simulink model "harness"  (Simulink 7.0)
settings: Solver=ode23  StartTime=0.0  StopTime=20  FixedStep=0.01  RelTol=1e-3
InitFcn:
  | init_simulation
StopFcn:
  | post_simulation
values from neighbouring files (symbols this model uses):
  A = pi*R^2    (= 0.0506707479097)    [constants.m]
  accel_noise = noise_on*.01^2    [constants.m]
  Alpha = pi/180*[-85:5:85]    [constants.m]
  att_noise = noise_on*(.25*pi/180)^2    [constants.m]
  att_ref = [0.2 0.2 0 0 0 0]'    [run_simulation.m]
  att_traj_on = 0    [set_scenario.m]
  b = 0.1    [constants.m]
  const_wind = [1 1 0]    [run_simulation.m]
  g = [0 0 9.8]'    [constants.m]
  gyro_noise = noise_on*.01^2    [constants.m]
  J = [Jxx 0 0 ... (first row only)    [constants.m]
  K_a1s = .009    (= 0.009)    [constants.m]
  K_attitude = [  0   kp_p   kp_y     0    kd_p   kd_y ... (first row only)    [run_simulation.m]
  K_beta = 0.23    [constants.m]
  K_dz = 0.7    [run_simulation.m]
  K_flap = 4*(K_beta + T_nom*dz)*K_a1s/(2*dx)    (= 0.0320793572835)    [constants.m]
  K_pz = .37    (= 0.37)    [run_simulation.m]
  K_torque = 0.47    [constants.m]
  M = 1.8263    [constants.m]
  motor_noise = noise_on*(9.8/4*.05)^2    [constants.m]
  plant_int_period = t_s / tau_motor    (= 0.00131578947368)    [constants.m]
  pos_noise = noise_on*0.02^2    [constants.m]
  r1 = [dx 0 -dz]'    [constants.m]
  r2 = [0 dx -dz]'    [constants.m]
  r3 = [-dx 0 -dz]'    [constants.m]
  r4 = [0 -dx -dz]'    [constants.m]
  R_90 = [0 -1 0 ... (first row only)    [constants.m]
  rho = 1.2    [constants.m]
  select = 0    [run_simulation.m]
  T_nom = M*9.8/4    (= 4.474435)    [constants.m]
  t_s = 1/76    (= 0.0131578947368)    [constants.m]
  tau_motor = 10    [constants.m]
  thrust_max = 9.8 * 1    (= 9.8)    [constants.m]
  thrust_min = 0    [constants.m]
  v_min = 1e-3    (= 0.001)    [constants.m]
  vel_noise = noise_on*0.05^2    [constants.m]
  Vh = sqrt(T/(2*rho*A))    [constants.m]
  Vinf = [0:0.5:6]    [constants.m]
  w_seed = 0    [run_simulation.m]
  wind = 3    [run_simulation.m]
  wind_clip = wind_max    (= 10)    [run_simulation.m]
  wind_duration = 5    [run_simulation.m]
  wind_max = 10    [run_simulation.m]
  wind_start = 3    [run_simulation.m]
  wind_var = (wind_max / 10)^2    (= 1)    [run_simulation.m]
  wind_vector = [1 0 0]'    [run_simulation.m]
  zd_ref = 0    [run_simulation.m]
undefined symbols (not defined in the file or in its folder): DiscIntNeverNeededParam, ToverTh
libraries: simulink x20
(part 3 of 3)

== system harness/Subsystem1/Aerodynamic Effects/Vertical Effect Dynamics/Motor 4 Vertical Effect Dynamics ==
  Thrust Command : Inport  OutDataType=sfix(16)  OutScaling=2^0
  V (body) : Inport  Port=2  OutDataType=sfix(16)  OutScaling=2^0
  Abs : Abs
  Constant : Constant  OutDataType=sfix(16)  OutScaling=2^0
  Demux : Demux  Outputs=3
  Divide : Product  Inputs=*/  OutDataType=sfix(16)  OutScaling=2^-10
  Dot Product : simulink/Math Operations/Dot Product  InputSameDT=on  OutDataType=sfix(16)  OutScaling=2^-10  DoSatur=off
  Math Function : Math  Operator=sqrt  OutDataType=sfix(16)  OutScaling=2^0  SaturateOnIntegerOverflow=on
  Saturation : Saturate  UpperLimit=500000  LowerLimit=0.00001
  Switch : Switch  Threshold=0.5
  T : Terminator
  T1 : Terminator
  TM1 : Scope
      settings: YMin=-1  YMax=11  SaveName=ScopeData18
  Trigonometric Function : Trigonometry  Operator=asin
  Unary Minus : simulink/Math Operations/Unary Minus  DoSatur=off
  alpha : Scope
      settings: YMin=0  YMax=1.75  SaveName=ScopeData17
  v_h : Scope
      settings: YMin=-1  YMax=11  SaveName=ScopeData15
  "v_h " : Fcn  Expr=sqrt(u/(2*rho*A))
  v_i Lookup Table (n-D) : Lookup_n-D  NumberOfTableDimensions=3  BreakpointsForDimension1=Alpha  BreakpointsForDimension2=Vinf  BreakpointsForDimension3=Vh  BeginIndexSearchUsingPreviousIndexResult=on  Table=ToverTh  InterpMethod=Cubic spline
  v_inf : Scope
      settings: YMin=-1  YMax=11  SaveName=ScopeData16
  Thrust Multiplier : Outport  OutDataType=sfix(16)  OutScaling=2^0
  wires:
  Thrust Command/1 -> "v_h "/1
  V (body)/1 -> Dot Product/1, Dot Product/2, Demux/1
  "v_h "/1 -> v_h/1, v_i Lookup Table (n-D)/3
  Dot Product/1 -> Math Function/1
  Math Function/1 -> v_inf/1, v_i Lookup Table (n-D)/2, Saturation/1  "v_inf"
  Demux/1 -> T/1
  Demux/2 -> T1/1
  Divide/1 -> Trigonometric Function/1
  Trigonometric Function/1 -> alpha/1, Abs/1, v_i Lookup Table (n-D)/1  "alpha"
  Switch/1 -> Thrust Multiplier/1
  v_i Lookup Table (n-D)/1 -> Switch/3, TM1/1
  Constant/1 -> Switch/1
  Abs/1 -> Switch/2
  Unary Minus/1 -> Divide/1
  Demux/3 -> Unary Minus/1
  Saturation/1 -> Divide/2
